simulink model "TestWCPS_v1"  (R2018a)
settings: Solver=VariableStepAuto  StartTime=0.0  StopTime=10.0  RelTol=1e-3
values from neighbouring files (symbols this model uses):
  A = [1.38 -0.2077 6.715 -5.676;-0.5814 -4.29 0 0.675;1.067 4.273 -6.654 5.893;0.048 4.273 1.343 -2.104]    [NCS_code.m]
  Ac = [0 0;0 0]    [NCS_code.m]
  B = [0 0;5.679 0;1.136 -3.146;1.136 0]    [NCS_code.m]
  Bc = [0 1;1 0]    [NCS_code.m]
  C = [1 0 1 -1;0 1 0 0]    [NCS_code.m]
  Cc = [2 0;0 -8]    [NCS_code.m]
  D = [0 0;0 0]    [NCS_code.m]
  Dc = [0 2;-5 0]    [NCS_code.m]
settings Model: Creator=root  LastModifiedBy=root

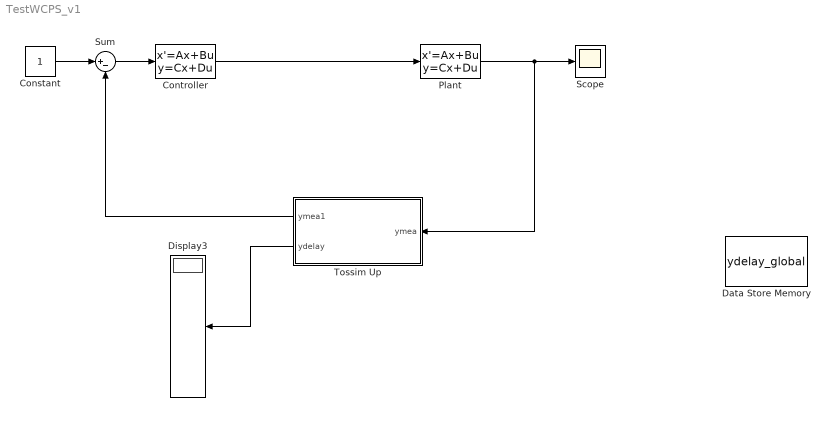
== system TestWCPS_v1 ==
  Constant : Constant
  Controller : StateSpace  A=Ac  B=Bc  C=Cc  D=Dc  InitialCondition=0
  Data Store Memory : DataStoreMemory  DataStoreName=ydelay_global  ReadBeforeWriteMsg=warning  WriteAfterWriteMsg=warning  WriteAfterReadMsg=warning  InitialValue=[1; 1; 1; 1; 1; 1; 1; 1; 1; 1; 1; 1; 1; 1; 1]  ShowAdditionalParam=off  OutDataTypeStr=uint32
  Display3 : Display
  Plant : StateSpace  A=A  B=B  C=C  D=D  InitialCondition=0
  Scope : Scope
  Sum : Sum  Inputs=|+-
  Tossim Up : MATLAB Function  TreatAsAtomicUnit=on
  wires:
  Plant/1 -> Tossim Up/1(ymea), Scope/1
  Controller/1 -> Plant/1
  Sum/1 -> Controller/1
  Constant/1 -> Sum/1
  Tossim Up/1(ymea1) -> Sum/2
  Tossim Up/2(ydelay) -> Display3/1

== matlab function TestWCPS_v1/Tossim Up ==
  settings: updateMethod=DISCRETE
  data: ymea1 output; ymea input; ydelay output; ydelay_global data_store_memory
function [ymea1, ydelay]  = Tossim_block(ymea)
% Inputs:
% ymea: measurement from structure
% Outputs:
% ymea1: measurement output
% ydelay: delay traces
persistent delay1 % delay trace
persistent i  % count
global ydelay_global


% allow these matlab functions to be used in Embedded Matlab block
eml.extrinsic('python');
eml.extrinsic('num2str');
eml.extrinsic('str2num');
eml.extrinsic('delay_summary');
eml.extrinsic('disp');
eml.extrinsic('ps_aggregation');
eml.extrinsic('for');
eml.extrinsic('end');

if isempty(i)
    i = 0;
end

ydelay = [1 0 0 0 0 0 0 0 0]';
% call python to communicate with TOSSIM

call_count = 18; %Superframelength
rssi = -69;%sensor rssi

[resultz] = ps_aggregation(call_count, rssi);%here call TOSSIM Client ----yh
end_to_end_delivery_result_aggregated = sum(resultz)

resultz

[delay] = delay_summary(end_to_end_delivery_result_aggregated);

delay

ydelay = delay';

delay1 = ydelay;
x =ydelay(2);
i = i+1;

ymea1 = ymea;

for i_yg = 1:9
    ydelay_global(i_yg, 1) = ydelay(i_yg, 1);
end
